simulink model "SOCPIControlBenchmarkRealVarL"  (R2019b)
settings: Solver=FixedStepAuto  StartTime=0.0  StopTime=50000  FixedStep=0.01  RelTol=1e-3
values from neighbouring files (symbols this model uses):
  kio = 0.6    [benchmarkPIDStartRealVarL.m]
  kpo = 1    [benchmarkPIDStartRealVarL.m]
  maxKi = 1    [benchmarkPIDStartRealVarL.m]
  maxKp = 1    [benchmarkPIDStartRealVarL.m]
  minKi = 0.01    [benchmarkPIDStartRealVarL.m]
  minKp = 0.01    [benchmarkPIDStartRealVarL.m]
  N = 100    [benchmarkPIDStartRealVarL.m]
  optimPeriod = 300    [benchmarkPIDStartRealVarL.m]
  OVLim = 2    [benchmarkPIDStartRealVarL.m]
  refAmplitude = 50    [benchmarkPIDStartRealVarL.m]
  refSignalPeriod = optimPeriod    (= 300)    [benchmarkPIDStartRealVarL.m]
  resetThreshold = 0.1    [benchmarkPIDStartRealVarL.m]
undefined symbols (not defined in the file or in its folder): FORandGCNM, sigbuilder_block
libraries: dspmathops x3, simulink x1
(part 1 of 4)
settings Model: Creator=jairo  LastModifiedBy=jairo
settings DataIOCC: ReturnWorkspaceOutputs=off

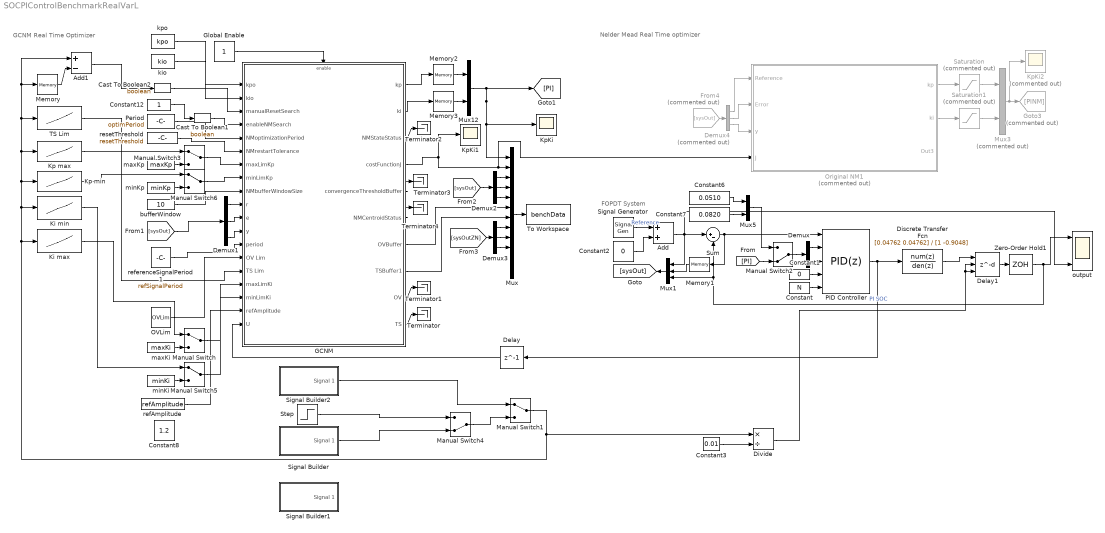
== system SOCPIControlBenchmarkRealVarL ==
  note: FOPDT System
  note: GCNM Real Time Optimizer
  note: Nelder Mead Real Time optimizer
  Add : Sum
  Add1 : Sum  Inputs=+-
  Cast To Boolean1 : DataTypeConversion  OutDataTypeStr=boolean
  Cast To Boolean2 : DataTypeConversion  OutDataTypeStr=boolean
  Constant : Constant  Value=N
  Constant1 : Constant  Value=0
  Constant12 : Constant  OutDataTypeStr=boolean
  Constant2 : Constant  Value=0
  Constant3 : Constant  Value=0.01
  Constant6 : Constant  Value=0.0510
  Constant7 : Constant  Value=0.0820
  Constant8 : Constant  Value=1.2
  Delay : Delay  DelayLength=1
  Delay1 : Delay  DelayLengthSource=Input port  DelayLengthUpperLimit=1000  InitialConditionSource=Input port
      settings: InputPortMap=u0,p1,p4
  Demux : Demux  Outputs=2
  Demux1 : Demux  Outputs=3
  Demux2 : Demux  Outputs=3
  Demux3 : Demux  Outputs=3
  Demux4 : Demux  Commented=on  Outputs=3
  Discrete Transfer Fcn : DiscreteTransferFcn  Numerator=[0.04762 0.04762]  Denominator=[1 -0.9048]
  Divide : Product  Inputs=*/
  From4 : From  Commented=on  GotoTag=sysOut
  GCNM : Subsystem
  Global Enable : Constant
  Goto3 : Goto  Commented=on  GotoTag=PINM
  Ki max : Lookup_n-D  NumberOfTableDimensions=1  BreakpointsForDimension1=[0.1 0.5 1 2 3 4 5 6 7 8 9 10]  UseOneInputPortForAllInputData=on  Table=|  InternalRulePriority=Speed  RndMeth=Simplest  InputSameDT=on
      | [11
      | 1.61
      | 0.9
      | 0.4
      | 0.4
      | 0.3
      | 0.18
      | 0.15
      | 0.12
      | 0.1
      | 0.09
      | 0.07]
  Ki min : Lookup_n-D  NumberOfTableDimensions=1  BreakpointsForDimension1=[0.1 0.5 1 2 3 4 5 6 7 8 9 10]  UseOneInputPortForAllInputData=on  Table=|  InternalRulePriority=Speed  RndMeth=Simplest  InputSameDT=on
      | [1.1
      | 0.41
      | 0.21
      | 0.21
      | 0.11
      | 0.11
      | 0.061
      | 0.06
      | 0.061
      | 0.061
      | 0.061
      | 0.041]
  Kp max : Lookup_n-D  NumberOfTableDimensions=1  BreakpointsForDimension1=[0.1 0.5 1 2 3 4 5 6 7 8 9 10]  UseOneInputPortForAllInputData=on  Table=|  InternalRulePriority=Speed  RndMeth=Simplest  InputSameDT=on
      | [16
      | 3.21
      | 1.8
      | 1
      | 1
      | 0.9
      | 0.68
      | 0.73
      | 0.69
      | 0.67
      | 0.63
      | 0.54]
  Kp min : Lookup_n-D  NumberOfTableDimensions=1  BreakpointsForDimension1=[0.1 0.5 1 2 3 4 5 6 7 8 9 10]  UseOneInputPortForAllInputData=on  Table=|  InternalRulePriority=Speed  RndMeth=Simplest  InputSameDT=on
      | [0.1
      | 0.01
      | 0.01
      | 0.01
      | 0.01
      | 0.01
      | 0.01
      | 0.01
      | 0.01
      | 0.01
      | 0.01
      | 0.01
      | ]
  KpKi : Scope
  KpKi1 : Scope
  KpKi2 : Scope  Commented=on
  Manual Switch{,1,3,5..6} (5 alike) : ManualSwitch
  Manual Switch2 : ManualSwitch  CurrentSetting=0
  Manual Switch4 : ManualSwitch  CurrentSetting=0
  Memory : Memory
  Memory1 : Memory
  Memory2 : Memory  InitialCondition=kpo
  Memory3 : Memory  InitialCondition=kio
  Mux : Mux  Inputs=12
  Mux1 : Mux  Inputs=3
  Mux12 : Mux  Inputs=2
  Mux3 : Mux  Commented=on  Inputs=2
  Mux5 : Mux  Inputs=2
  OVLim : Constant  Value=OVLim
  Original NM1 : Subsystem  Commented=on
  PID Controller : simulink/Continuous/PID Controller  Controller=PID  Form=Parallel  TimeDomain=Discrete-time  SampleTime=0.1  IntegratorMethod=Forward Euler  FilterMethod=Forward Euler  ControllerParametersSource=external  P=1  I=100  D=0  UseFilter=on  N=100  TunerSelectOption=Transfer Function Based (PID Tuner App)  InitialConditionSource=internal  InitialConditionForIntegrator=0  InitialConditionForFilter=0  DifferentiatorICPrevScaledInput=0  ExternalReset=none  TrackingMode=off  Kt=1  LimitOutput=off  UpperSaturationLimit=inf  LowerSaturationLimit=-inf  LinearizeAsGain=on  AntiWindupMode=none  Kb=1  POutMin=[]  POutMax=[]  IOutMin=[]  IOutMax=[]  DOutMin=[]  DOutMax=[]  NOutMin=[]  NOutMax=[]  SumOutMin=[]  SumOutMax=[]  SaturationOutMin=[]  SaturationOutMax=[]  PParamMin=[]  PParamMax=[]  IParamMin=[]  IParamMax=[]  DParamMin=[]  DParamMax=[]  NParamMin=[]  NParamMax=[]  KbParamMin=[]  KbParamMax=[]  KtParamMin=[]  KtParamMax=[]  KbOutMin=[]  KbOutMax=[]  KtOutMin=[]  KtOutMax=[]  IntegratorOutMin=[]  IntegratorOutMax=[]  FilterOutMin=[]  FilterOutMax=[]  SumI1OutMin=[]  SumI1OutMax=[]  SumI2OutMin=[]  SumI2OutMax=[]  SumI3OutMin=[]  SumI3OutMax=[]  SumI4OutMin=[]  SumI4OutMax=[]  SumDOutMin=[]  SumDOutMax=[]  DifferentiatorOutMin=[]  DifferentiatorOutMax=[]  FilterDiffOutCoefMin=[]  FilterDiffOutCoefMax=[]  ReciprocalOutMin=[]  ReciprocalOutMax=[]  SumDenOutMin=[]  SumDenOutMax=[]  SumNumOutMin=[]  SumNumOutMax=[]  DivideOutMin=[]  DivideOutMax=[]  IntegratorContinuousStateAttributes=''  IntegratorStateMustResolveToSignalObject=off  IntegratorRTWStateStorageClass=Auto  FilterContinuousStateAttributes=''  FilterStateMustResolveToSignalObject=off  FilterRTWStateStorageClass=Auto  ParallelPVariant=ExternalParameters  IdealPVariant=Disabled  IVariant=ExternalParameters  DVariant=ExternalParameters  IntegratorVariant=Discrete  SatVariant=Disabled  AWVariant=Passthrough  PCopyVariant=Disabled  TRVariant=Disabled  FdbkBlocksVariant=Forward  IdealPFdbkVariant=Disabled  SatFdbkVariant=Disabled  DerivativeFilterVariant=ForwardEulerFilter  NVariant=ExternalParameters  NCopyVariant=Disabled  FilterICVariant=InternalICsFilter  IntegratorICVariant=InternalICs  ExternalResetVariant=Disabled  TRSumVariant=Passthrough  SumFdbkVariant=Disabled  SumVariant=Sum_PID
  Period : Constant  Value=optimPeriod  OutDataTypeStr=double
  Saturation : Saturate  Commented=on  UpperLimit=maxKp  LowerLimit=minKp
  Saturation1 : Saturate  Commented=on  UpperLimit=maxKi  LowerLimit=minKi
  Signal Generator : SignalGenerator  WaveForm=square  Frequency=1/refSignalPeriod
  Signal Builder : Subsystem  Tag=STV Subsys  LoadFcn=sigbuilder_block('load');  StartFcn=sigbuilder_block('start');  StopFcn=sigbuilder_block('stop');  ClipboardFcn=sigbuilder_block('clipboard');  mask(Sigbuilder block){tuvar=[0:10]}
      mask help: Simulink:masks:SigbuilderBlock_MD
      mask init:
      | if ~strcmp(get_param(bdroot(gcbh),'SimulationStatus'),'stopped') tuvar = sigbuilder_block('maskInit'); end
      settings: CopyFcn=sigbuilder_block('copy');  DeleteFcn=sigbuilder_block('delete');  ModelCloseFcn=sigbuilder_block('modelClose');  PreSaveFcn=sigbuilder_block('preSave');  PauseFcn=sigbuilder_block('pause');  ContinueFcn=sigbuilder_block('continue');  NameChangeFcn=sigbuilder_block('namechange');  OpenFcn=sigbuilder_block('open',[5.4 30.6 1141.2 522.6 ]);  CloseFcn=sigbuilder_block('close');
      mask Display: plot(0, 0, 100, 100,[2, 2, 32, 32, 2], [68, 8, 8, 68, 68],[32, 2], [38, 38], [32, 19, 2],[53, 60, 44], [32, 17, 17, 2],[16, 16, 31, 31]);txt = getActiveGroup(gcbh);text(2, 100, txt,'verticalAlignment', 'top');
  Signal Builder1 : Subsystem  Tag=STV Subsys  LoadFcn=sigbuilder_block('load');  StartFcn=sigbuilder_block('start');  StopFcn=sigbuilder_block('stop');  ClipboardFcn=sigbuilder_block('clipboard');  mask(Sigbuilder block){tuvar=[0:10]}
      mask help: Simulink:masks:SigbuilderBlock_MD
      mask init:
      | if ~strcmp(get_param(bdroot(gcbh),'SimulationStatus'),'stopped') tuvar = sigbuilder_block('maskInit'); end
      settings: CopyFcn=sigbuilder_block('copy');  DeleteFcn=sigbuilder_block('delete');  ModelCloseFcn=sigbuilder_block('modelClose');  PreSaveFcn=sigbuilder_block('preSave');  PauseFcn=sigbuilder_block('pause');  ContinueFcn=sigbuilder_block('continue');  NameChangeFcn=sigbuilder_block('namechange');  OpenFcn=sigbuilder_block('open',[5.4 30.6 1141.2 522.6 ]);  CloseFcn=sigbuilder_block('close');
      mask Display: plot(0, 0, 100, 100,[2, 2, 32, 32, 2], [68, 8, 8, 68, 68],[32, 2], [38, 38], [32, 19, 2],[53, 60, 44], [32, 17, 17, 2],[16, 16, 31, 31]);txt = getActiveGroup(gcbh);text(2, 100, txt,'verticalAlignment', 'top');
  Signal Builder2 : Subsystem  Tag=STV Subsys  LoadFcn=sigbuilder_block('load');  StartFcn=sigbuilder_block('start');  StopFcn=sigbuilder_block('stop');  ClipboardFcn=sigbuilder_block('clipboard');  mask(Sigbuilder block){tuvar=[0:10]}
      mask help: Simulink:masks:SigbuilderBlock_MD
      mask init:
      | if ~strcmp(get_param(bdroot(gcbh),'SimulationStatus'),'stopped') tuvar = sigbuilder_block('maskInit'); end
      settings: CopyFcn=sigbuilder_block('copy');  DeleteFcn=sigbuilder_block('delete');  ModelCloseFcn=sigbuilder_block('modelClose');  PreSaveFcn=sigbuilder_block('preSave');  PauseFcn=sigbuilder_block('pause');  ContinueFcn=sigbuilder_block('continue');  NameChangeFcn=sigbuilder_block('namechange');  OpenFcn=sigbuilder_block('open',[5.4 30.6 1141.2 522.6 ]);  CloseFcn=sigbuilder_block('close');
      mask Display: plot(0, 0, 100, 100,[2, 2, 32, 32, 2], [68, 8, 8, 68, 68],[32, 2], [38, 38], [32, 19, 2],[53, 60, 44], [32, 17, 17, 2],[16, 16, 31, 31]);txt = getActiveGroup(gcbh);text(2, 100, txt,'verticalAlignment', 'top');
  Step : Step  Time=21000  Before=0.1  After=5  SampleTime=0
  Sum : Sum  Inputs=|+-
  TS Lim : Lookup_n-D  NumberOfTableDimensions=1  BreakpointsForDimension1=[0.1 0.5 1 2 3 4 5 6 7 8 9 10]  UseOneInputPortForAllInputData=on  Table=|  InternalRulePriority=Speed  RndMeth=Simplest  InputSameDT=on
      | [40
      | 40
      | 100
      | 100
      | 100
      | 100
      | 100
      | 100
      | 100
      | 100
      | 100
      | 100]
  Terminator{,1..4} (5 alike) : Terminator
  To Workspace : ToWorkspace  VariableName=benchData  SaveFormat=Timeseries  SampleTime=-1
  Zero-Order Hold1 : ZeroOrderHold  SampleTime=-1
  bufferWindow : Constant  Value=10  OutDataTypeStr=uint16
  kio : Constant  Value=kio  OutDataTypeStr=double
  kpo : Constant  Value=kpo  OutDataTypeStr=double
  maxKi : Constant  Value=maxKi  VectorParams1D=off  OutDataTypeStr=double
  maxKp : Constant  Value=maxKp  OutDataTypeStr=double
  minKi : Constant  Value=minKi  OutDataTypeStr=double
  minKp : Constant  Value=minKp  OutDataTypeStr=double
  output : Scope  NumInputPorts=3
  refAmplitude : Constant  Value=refAmplitude  OutDataTypeStr=double
  referenceSignalPeriod1 : Constant  Value=refSignalPeriod
  resetThreshold : Constant  Value=resetThreshold
  wires:
  PID Controller/1 -> Discrete Transfer Fcn/1, Delay/1
  Sum/1 -> Memory1/1, PID Controller/1
  resetThreshold/1 -> GCNM/6(NMrestartTolerance)
  bufferWindow/1 -> GCNM/9(NMbufferWindowSize)
  Cast To Boolean1/1 -> GCNM/4(enableNMSearch)
  kio/1 -> GCNM/2(kio)
  Constant12/1 -> Cast To Boolean1/1
  Global Enable/1 -> GCNM/Enable
  kpo/1 -> GCNM/1(kpo)
  Period/1 -> GCNM/5(NMoptimizationPeriod)
  GCNM/4(costFunctionJ) -> Original NM1/4(J), Mux/2, KpKi1/1
  OVLim/1 -> GCNM/14("  OV Lim")
  Zero-Order Hold1/1 -> output/1, Sum/2, Mux1/3  "PI SOC"
  GCNM/1("  kp") -> Memory2/1
  GCNM/2("  ki") -> Memory3/1
  Mux/1 -> To Workspace/1
  Constant/1 -> PID Controller/5
  Constant1/1 -> PID Controller/4
  Demux/1 -> PID Controller/2
  Demux/2 -> PID Controller/3
  Mux1/1 -> [sysOut]
  [sysOut] -> Demux1/1
  Demux1/1 -> GCNM/10(r)
  Demux1/2 -> GCNM/11("  e")
  Demux1/3 -> GCNM/12("  y")
  [sysOut] -> Demux2/1
  Demux2/1 -> Mux/3
  Demux2/2 -> Mux/4
  Demux2/3 -> Mux/5
  [sysOutZN] -> Demux3/1
  Demux3/1 -> Mux/8
  Demux3/2 -> Mux/9
  Demux3/3 -> Mux/10
  Demux4/2 -> Original NM1/2(Error)
  Demux4/3 -> Original NM1/3(y)
  From4/1 -> Demux4/1
  Demux4/1 -> Original NM1/1(Reference)
  GCNM/10(TS) -> Terminator/1
  GCNM/9(OV) -> Terminator1/1
  GCNM/8(TSBuffer1) -> Mux/7
  GCNM/7(OVBuffer) -> Mux/6
  GCNM/3(NMStateStatus) -> Terminator2/1
  GCNM/5(convergenceThresholdBuffer) -> Terminator3/1
  GCNM/6(NMCentroidStatus) -> Terminator4/1
  Signal Generator/1 -> Add/1  "Reference"
  Constant2/1 -> Add/2
  Add/1 -> output/3, Mux1/1, Sum/1
  refAmplitude/1 -> GCNM/18(refAmplitude)
  Manual Switch2/1 -> Demux/1
  [PI] -> Manual Switch2/2
  Original NM1/2(ki) -> Saturation1/1
  Original NM1/1(kp) -> Saturation/1
  Mux3/1 -> KpKi2/1, Goto3/1
  Mux5/1 -> Manual Switch2/1
  Saturation/1 -> Mux3/1
  Saturation1/1 -> Mux3/2
  Delay/1 -> GCNM/19("  U")
  maxKi/1 -> Manual Switch/2
  Manual Switch/1 -> GCNM/16(maxLimKi)
  Manual Switch3/1 -> GCNM/7(maxLimKp)
  maxKp/1 -> Manual Switch3/2
  Step/1 -> Manual Switch4/1
  Signal Builder/1(Signal 1) -> Manual Switch4/2
  Manual Switch4/1 -> Manual Switch1/2
  minKi/1 -> Manual Switch5/2
  minKp/1 -> Manual Switch6/2
  Manual Switch6/1 -> GCNM/8(minLimKp)
  Manual Switch5/1 -> GCNM/17(minLimKi)
  Divide/1 -> Delay1/3, Delay1/2
  Constant3/1 -> Divide/2
  Discrete Transfer Fcn/1 -> Delay1/1
  Delay1/1 -> Zero-Order Hold1/1
  Mux12/1 -> KpKi/1, Mux/1, [PI]
  Memory1/1 -> Mux1/2
  Memory2/1 -> Mux12/1
  Memory3/1 -> Mux12/2
  Constant7/1 -> Mux5/2
  Constant6/1 -> Mux5/1
  Kp max/1 -> Manual Switch3/1
  Kp min/1 -> Manual Switch6/1
  Ki max/1 -> Manual Switch/1
  Ki min/1 -> Manual Switch5/1
  TS Lim/1 -> GCNM/15(TS Lim)
  referenceSignalPeriod1/1 -> GCNM/13("  period")
  Manual Switch1/1 -> Divide/1, Add1/1, Memory/1, TS Lim/1, Kp max/1, Kp min/1, Ki min/1, Ki max/1
  Memory/1 -> Add1/2
  Add1/1 -> Cast To Boolean2/1
  Cast To Boolean2/1 -> GCNM/3(manualResetSearch)
  Signal Builder2/1(Signal 1) -> Manual Switch1/1

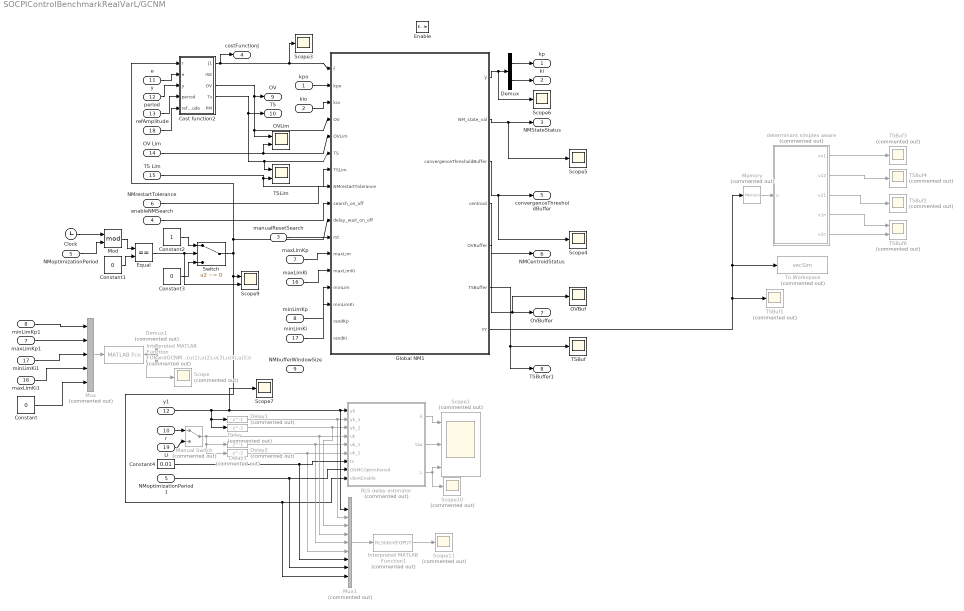
== system SOCPIControlBenchmarkRealVarL/GCNM ==
  kpo : Inport  OutDataTypeStr=double
  kio : Inport  Port=2  OutDataTypeStr=double
  manualResetSearch : Inport  Port=3  OutDataTypeStr=boolean
  enableNMSearch : Inport  Port=4  OutDataTypeStr=boolean
  NMoptimizationPeriod : Inport  Port=5  OutDataTypeStr=double
  NMrestartTolerance : Inport  Port=6
  maxLimKp : Inport  Port=7  OutDataTypeStr=double
  minLimKp : Inport  Port=8  OutDataTypeStr=double
  NMbufferWindowSize : Inport  Port=9  OutDataTypeStr=uint16
  r : Inport  Port=10
  "  e" : Inport  Port=11  OutDataTypeStr=double
  "  y" : Inport  Port=12  OutDataTypeStr=double
  "  period" : Inport  Port=13  OutDataTypeStr=double
  "  OV Lim" : Inport  Port=14  OutDataTypeStr=double
  TS Lim : Inport  Port=15  OutDataTypeStr=double
  maxLimKi : Inport  Port=16  OutDataTypeStr=double
  minLimKi : Inport  Port=17  OutDataTypeStr=double
  refAmplitude : Inport  Port=18  OutDataTypeStr=double
  "  U" : Inport  Port=19  OutDataTypeStr=double
  Enable : EnablePort
  "  y1" : InportShadow  Port=12  OutDataTypeStr=double
  Clock : Clock
  Constant : Constant  Value=0
  Constant1 : Constant  Value=0
  Constant2 : Constant
  Constant3 : Constant  Value=0
  Constant4 : Constant  Value=0.01
  Cost function2 : Subsystem
  Delay : Delay  Commented=on
  Delay1 : Delay  Commented=on  DelayLength=1
  Delay2 : Delay  Commented=on
  Delay3 : Delay  Commented=on  DelayLength=1
  Demux : Demux  Outputs=2
  Demux1 : Demux  Commented=on  Outputs=2
  Equal : RelationalOperator  Operator===  RndMeth=Simplest
  Global NM1 : MATLAB Function  TreatAsAtomicUnit=on
  Interpreted MATLAB Function : MATLABFcn  Commented=on  MATLABFcn=FORandGCNM(u(1),u(2),u(3),u(4),u(5))  OutputDimensions=2
  Interpreted MATLAB Function1 : MATLABFcn  Commented=on  MATLABFcn=RLSIdentFOPDT  OutputDimensions=3
  Manual Switch : ManualSwitch  Commented=on
  Memory : Memory  Commented=on
  Mod : Math  Operator=mod  SignedPower=off  SaturateOnIntegerOverflow=on
  Mux : Mux  Commented=on  Inputs=5
  Mux1 : Mux  Commented=on  Inputs=9
  NMoptimizationPeriod1 : InportShadow  Port=5  OutDataTypeStr=double
  OVBuf : Scope
  OVLim : Scope  NumInputPorts=2
  RLS delay estimator : MATLAB Function  Commented=on  TreatAsAtomicUnit=on  SystemSampleTime=0.01
  Scope : Scope  Commented=on
  Scope1 : Scope  Commented=on  NumInputPorts=3
  Scope10 : Scope  Commented=on
  Scope11 : Scope  Commented=on
  Scope{3..7} (5 alike) : Scope
  Scope9 : Scope  NumInputPorts=2
  Switch : Switch  Criteria=u2 ~= 0
  TSBuf : Scope
  TSBuf{1..4} (4 alike) : Scope  Commented=on
  TSBuf6 : Scope  Commented=on  NumInputPorts=2
  TSLim : Scope  NumInputPorts=2
  To Workspace : ToWorkspace  Commented=on  VariableName=vecSim  SampleTime=-1
  determinant simplex aware : MATLAB Function  Commented=on  TreatAsAtomicUnit=on
  maxLimKi1 : InportShadow  Port=16  OutDataTypeStr=double
  maxLimKp1 : InportShadow  Port=7  OutDataTypeStr=double
  minLimKi1 : InportShadow  Port=17  OutDataTypeStr=double
  minLimKp1 : InportShadow  Port=8  OutDataTypeStr=double
  "  kp" : Outport  OutDataTypeStr=double
  "  ki" : Outport  Port=2  OutDataTypeStr=double
  NMStateStatus : Outport  Port=3  OutDataTypeStr=double
  costFunctionJ : Outport  Port=4  OutDataTypeStr=double
  convergenceThresholdBuffer : Outport  Port=5  OutDataTypeStr=double
  NMCentroidStatus : Outport  Port=6  OutDataTypeStr=double
  OVBuffer : Outport  Port=7  OutDataTypeStr=double
  TSBuffer1 : Outport  Port=8  OutDataTypeStr=double
  OV : Outport  Port=9  OutDataTypeStr=double
  TS : Outport  Port=10  OutDataTypeStr=double
  wires:
  Demux/2 -> "  ki"/1
  Demux/1 -> "  kp"/1
  NMrestartTolerance/1 -> Global NM1/8(NMrestartTolerance)
  manualResetSearch/1 -> Global NM1/11(rst)
  enableNMSearch/1 -> Global NM1/9(search_on_off)
  minLimKp/1 -> Global NM1/14(minLim)
  maxLimKp/1 -> Global NM1/12(maxLim)
  Global NM1/2(NM_state_val) -> Scope5/1, NMStateStatus/1
  Global NM1/3(convergenceThresholdBuffer) -> convergenceThresholdBuffer/1, Scope4/1
  Global NM1/4(centroid) -> NMCentroidStatus/1
  Global NM1/1(y) -> Scope6/1, Demux/1
  kpo/1 -> Global NM1/2(kpo)
  kio/1 -> Global NM1/3(kio)
  Cost function2/3(OV) -> OV/1, Global NM1/4(OV), OVLim/1
  "  y"/1 -> Cost function2/3(y)
  "  e"/1 -> Cost function2/2(e)
  Global NM1/5(OVBuffer) -> OVBuf/1, OVBuffer/1
  "  period"/1 -> Cost function2/4(period)
  "  OV Lim"/1 -> OVLim/2, Global NM1/5(OVLim)
  Cost function2/4(Ts) -> TS/1, Global NM1/6(TS), TSLim/1
  TS Lim/1 -> Global NM1/7(TSLim), TSLim/2
  Global NM1/6(TSBuffer) -> TSBuffer1/1, TSBuf/1
  Cost function2/1(J1) -> Scope3/1, Global NM1/1(f), costFunctionJ/1
  Clock/1 -> Mod/1
  NMoptimizationPeriod/1 -> Mod/2
  Constant1/1 -> Equal/2
  Mod/1 -> Equal/1
  Constant2/1 -> Switch/1
  Constant3/1 -> Switch/3
  Switch/1 -> Mux1/9, RLS delay estimator/9(identEnable), Scope9/1, Cost function2/1(r), Global NM1/10(delay_wait_on_off)
  Equal/1 -> Scope9/2, Switch/2
  maxLimKi/1 -> Global NM1/13(maxLimKi)
  minLimKi/1 -> Global NM1/15(minLimKi)
  refAmplitude/1 -> Cost function2/5(refAmplitude)
  minLimKi1/1 -> Mux/3
  maxLimKi1/1 -> Mux/4
  Mux/1 -> Interpreted MATLAB Function/1
  Interpreted MATLAB Function/1 -> Scope/1, Demux1/1
  maxLimKp1/1 -> Mux/2
  minLimKp1/1 -> Mux/1
  Constant/1 -> Mux/5
  determinant simplex aware/2(v12) -> TSBuf4/1
  Memory/1 -> determinant simplex aware/1(u)
  Global NM1/7(YY) -> TSBuf1/1, To Workspace/1, Memory/1
  determinant simplex aware/5(v2n) -> TSBuf6/2
  determinant simplex aware/3(v21) -> TSBuf2/1
  determinant simplex aware/4(v1n) -> TSBuf6/1
  determinant simplex aware/1(vv1) -> TSBuf3/1
  Delay1/1 -> Mux1/2, RLS delay estimator/2(yk_1)
  Delay/1 -> Mux1/3, RLS delay estimator/3(yk_2)
  "  y1"/1 -> Delay1/1, Delay/1, Scope7/1, Mux1/1, RLS delay estimator/1(yk)
  Delay3/1 -> Mux1/5, RLS delay estimator/5(uk_1)
  Delay2/1 -> RLS delay estimator/6(uk_2), Mux1/6
  NMoptimizationPeriod1/1 -> Mux1/8, RLS delay estimator/8(GNMCOptimPeriod)
  RLS delay estimator/1(k) -> Scope1/1
  RLS delay estimator/2(tau) -> Scope1/2
  RLS delay estimator/3(L) -> Scope1/3, Scope10/1
  Constant4/1 -> Mux1/7, RLS delay estimator/7(ts)
  r/1 -> Manual Switch/1
  "  U"/1 -> Manual Switch/2
  Manual Switch/1 -> Mux1/4, RLS delay estimator/4(uk), Delay2/1, Delay3/1
  Mux1/1 -> Interpreted MATLAB Function1/1
  Interpreted MATLAB Function1/1 -> Scope11/1

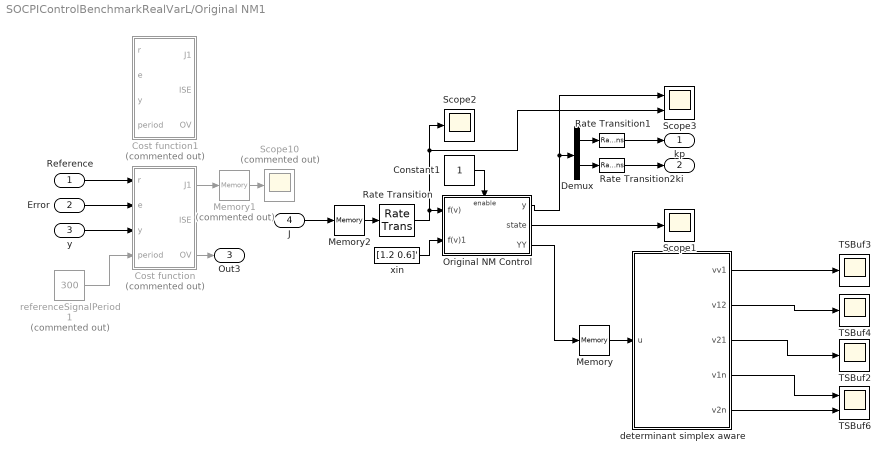
== system SOCPIControlBenchmarkRealVarL/Original NM1 ==
  Reference : Inport
  Error : Inport  Port=2
  y : Inport  Port=3
  J : Inport  Port=4
  Constant1 : Constant
  Cost function : Subsystem  Commented=on
  Cost function1 : Subsystem  Commented=on
  Demux : Demux  Outputs=2
  Memory : Memory
  Memory1 : Memory  Commented=on
  Memory2 : Memory
  Original NM Control : Subsystem
  Rate Transition : RateTransition
  Rate Transition1 : RateTransition  InitialCondition=1
  Rate Transition2 : RateTransition  InitialCondition=100
  Scope1 : Scope
  Scope10 : Scope  Commented=on
  Scope2 : Scope
  Scope3 : Scope  NumInputPorts=2
  TSBuf2 : Scope
  TSBuf3 : Scope
  TSBuf4 : Scope
  TSBuf6 : Scope  NumInputPorts=2
  determinant simplex aware : MATLAB Function  TreatAsAtomicUnit=on
  referenceSignalPeriod1 : Constant  Commented=on  Value=300
  xin : Constant  Value=[1.2 0.6]'
  kp : Outport
  ki : Outport  Port=2
  Out3 : Outport  Port=3
  wires:
  Constant1/1 -> Original NM Control/Enable
  Original NM Control/1(y) -> Scope3/1, Demux/1
  Rate Transition/1 -> Scope2/1, Scope3/2, Original NM Control/1(f(v))
  Demux/2 -> Rate Transition2/1
  xin/1 -> Original NM Control/2(f(v)1)
  y/1 -> Cost function/3(y)
  Original NM Control/2(state) -> Scope1/1
  Demux/1 -> Rate Transition1/1
  Memory2/1 -> Rate Transition/1
  Cost function/3(OV) -> Out3/1
  Memory1/1 -> Scope10/1
  referenceSignalPeriod1/1 -> Cost function/4(period)
  Cost function/1(J1) -> Memory1/1
  Rate Transition1/1 -> kp/1
  Rate Transition2/1 -> ki/1
  Reference/1 -> Cost function/1(r)
  Error/1 -> Cost function/2(e)
  J/1 -> Memory2/1
  determinant simplex aware/2(v12) -> TSBuf4/1
  determinant simplex aware/5(v2n) -> TSBuf6/2
  determinant simplex aware/4(v1n) -> TSBuf6/1
  determinant simplex aware/1(vv1) -> TSBuf3/1
  determinant simplex aware/3(v21) -> TSBuf2/1
  Memory/1 -> determinant simplex aware/1(u)
  Original NM Control/3(YY) -> Memory/1

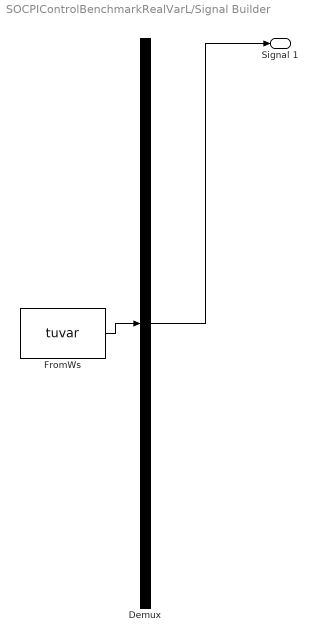
== system SOCPIControlBenchmarkRealVarL/Signal Builder ==
  Demux : Demux  Tag=STV Demux  Outputs=1
  FromWs : FromWorkspace  Tag=STV FromWs  VariableName=tuvar  SampleTime=0
      SigBuilderData=|
      | common.afterFinalStr = 'Extrapolate'
      | common.sampleTime = 0
      | dataSet.timeRange = [0 50000]
      | dataSet.name = 'Group 1'
      | sbobj.Groups.Name = 'Group 1'
      | sbobj.Groups.Signals.Name = 'Signal 1'
      | sbobj.Groups.Signals.XData = [0 12000 12000 21000 21000 36000 36000 50000]
      | sbobj.Groups.Signals.YData = [0.1 0.1 5 5 8 8 3 3]
      | sbobj.Groups.TimeRange = [0 50000]
  Signal 1 : Outport  Tag=STV Outport
  wires:
  Demux/1 -> Signal 1/1
  FromWs/1 -> Demux/1

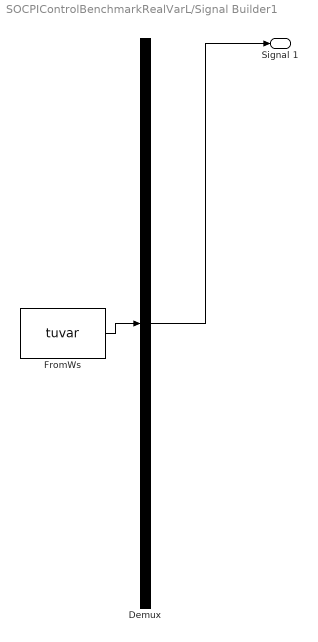
== system SOCPIControlBenchmarkRealVarL/Signal Builder1 ==
  Demux : Demux  Tag=STV Demux  Outputs=1
  FromWs : FromWorkspace  Tag=STV FromWs  VariableName=tuvar  SampleTime=0
      SigBuilderData=|
      | common.afterFinalStr = 'Extrapolate'
      | common.sampleTime = 0
      | dataSet.timeRange = [0 50000]
      | dataSet.name = 'Group 1'
      | sbobj.Groups.Name = 'Group 1'
      | sbobj.Groups.Signals.Name = 'Signal 1'
      | sbobj.Groups.Signals.XData = [0 12000 12000 21000 21000 36000 36000 50000]
      | sbobj.Groups.Signals.YData = [7.98 7.98 5.86 5.86 0.64 0.64 4.2 4.2]
      | sbobj.Groups.TimeRange = [0 50000]
  Signal 1 : Outport  Tag=STV Outport
  wires:
  FromWs/1 -> Demux/1
  Demux/1 -> Signal 1/1

== system SOCPIControlBenchmarkRealVarL/Signal Builder2 ==
  Demux : Demux  Tag=STV Demux  Outputs=1
  FromWs : FromWorkspace  Tag=STV FromWs  VariableName=tuvar  SampleTime=0
      SigBuilderData=|
      | common.afterFinalStr = 'Extrapolate'
      | common.sampleTime = 0
      | dataSet.timeRange = [0 50000]
      | dataSet.name = 'Group 1'
      | sbobj.Groups.Name = 'Group 1'
      | sbobj.Groups.Signals.Name = 'Signal 1'
      | sbobj.Groups.Signals.XData = [0 10050 10050 21000 21000 36000 36000 50000]
      | sbobj.Groups.Signals.YData = [0.1 0.1 9 9 5 5 1 1]
      | sbobj.Groups.TimeRange = [0 50000]
  Signal 1 : Outport  Tag=STV Outport
  wires:
  Demux/1 -> Signal 1/1
  FromWs/1 -> Demux/1

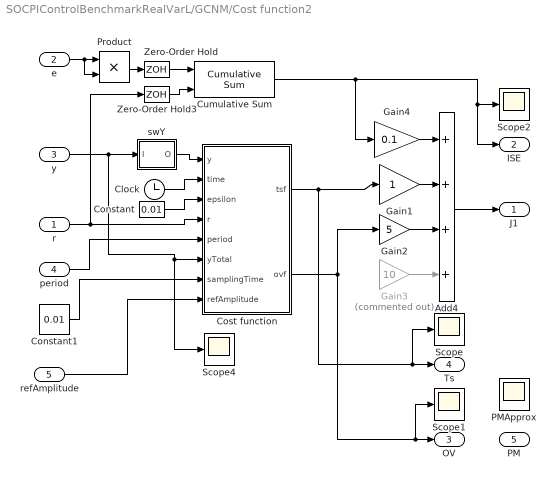
== system SOCPIControlBenchmarkRealVarL/GCNM/Cost function2 ==
  r : Inport
  e : Inport  Port=2
  y : Inport  Port=3
  period : Inport  Port=4
  refAmplitude : Inport  Port=5
  Add4 : Sum  Inputs=++++
  Clock : Clock
  Constant : Constant  Value=0.01
  Constant1 : Constant  Value=0.01
  Cost function : MATLAB Function  TreatAsAtomicUnit=on
  Cumulative Sum : dspmathops/Cumulative Sum  dim=Channels (running sum)  InputProcessing=Columns as channels (frame based)  reset_popup=Falling edge  roundingMode=Floor  overflowMode=off  outputDataTypeStr=Inherit: Same as accumulator  outputMin=[]  outputMax=[]  outputLastDataTypeStr=Inherit: Same as accumulator
      settings: SourceProductName=DSP System Toolbox
  Gain1 : Gain
  Gain2 : Gain  Gain=5
  Gain3 : Gain  Commented=on  Gain=10
  Gain4 : Gain  Gain=0.1
  PMApprox : Scope
  Product : Product
  Scope{,1..2,4} (4 alike) : Scope
  Zero-Order Hold : ZeroOrderHold  SampleTime=-1
  Zero-Order Hold3 : ZeroOrderHold  SampleTime=-1
  swY : Subsystem
  J1 : Outport
  ISE : Outport  Port=2
  OV : Outport  Port=3
  Ts : Outport  Port=4
  PM : Outport  Port=5
  wires:
  Cumulative Sum/1 -> Gain4/1, ISE/1, Scope2/1
  Zero-Order Hold3/1 -> Cumulative Sum/2
  e/1 -> Product/2, Product/1
  Zero-Order Hold/1 -> Cumulative Sum/1
  r/1 -> Zero-Order Hold3/1, Cost function/4(r)
  swY/1(O) -> Cost function/1(y)
  Clock/1 -> Cost function/2(time)
  Product/1 -> Zero-Order Hold/1
  Constant/1 -> Cost function/3(epsilon)
  y/1 -> Scope4/1, Cost function/6(yTotal), swY/1(I)
  Add4/1 -> J1/1
  Gain2/1 -> Add4/3
  period/1 -> Cost function/5(period)
  Constant1/1 -> Cost function/7(samplingTime)
  Gain1/1 -> Add4/2
  refAmplitude/1 -> Cost function/8(refAmplitude)
  Gain3/1 -> Add4/4
  Cost function/1(tsf) -> Gain1/1, Scope/1, Ts/1
  Cost function/2(ovf) -> Gain2/1, Scope1/1, OV/1
  Gain4/1 -> Add4/1

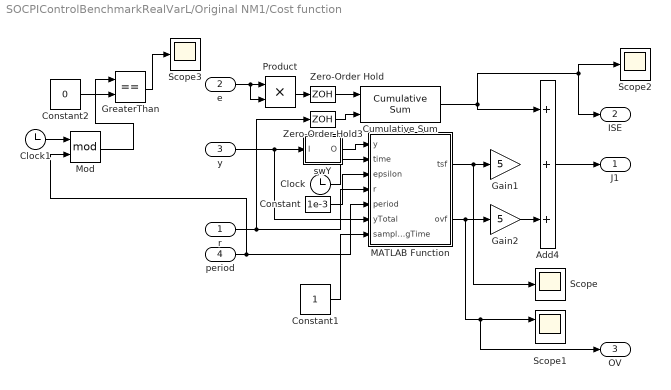
== system SOCPIControlBenchmarkRealVarL/Original NM1/Cost function ==
  r : Inport
  e : Inport  Port=2
  y : Inport  Port=3
  period : Inport  Port=4
  Add4 : Sum  Inputs=+++
  Clock : Clock
  Clock1 : Clock
  Constant : Constant  Value=1e-3
  Constant1 : Constant
  Constant2 : Constant  Value=0
  Cumulative Sum : dspmathops/Cumulative Sum  dim=Channels (running sum)  InputProcessing=Columns as channels (frame based)  reset_popup=Falling edge  roundingMode=Floor  overflowMode=off  outputDataTypeStr=Inherit: Same as accumulator  outputMin=[]  outputMax=[]  outputLastDataTypeStr=Inherit: Same as accumulator
      settings: SourceProductName=DSP System Toolbox
  Gain1 : Gain  Gain=5
  Gain2 : Gain  Gain=5
  GreaterThan : RelationalOperator  Operator===  OutDataTypeStr=boolean  RndMeth=Simplest
  MATLAB Function : MATLAB Function  TreatAsAtomicUnit=on
  Mod : Math  Operator=mod  SignedPower=off  SaturateOnIntegerOverflow=on
  Product : Product
  Scope : Scope
  Scope1 : Scope  NumInputPorts=2
  Scope2 : Scope
  Scope3 : Scope
  Zero-Order Hold : ZeroOrderHold  SampleTime=-1
  Zero-Order Hold3 : ZeroOrderHold  SampleTime=-1
  swY : Subsystem
  J1 : Outport
  ISE : Outport  Port=2
  OV : Outport  Port=3
  wires:
  Cumulative Sum/1 -> Add4/1, ISE/1, Scope2/1
  Zero-Order Hold3/1 -> Cumulative Sum/2
  e/1 -> Product/2, Product/1
  MATLAB Function/1(tsf) -> Scope/1, Gain1/1
  Zero-Order Hold/1 -> Cumulative Sum/1
  r/1 -> Zero-Order Hold3/1, MATLAB Function/4(r)
  MATLAB Function/2(ovf) -> OV/1, Scope1/1, Gain2/1
  swY/1(O) -> MATLAB Function/1(y)
  Clock/1 -> MATLAB Function/2(time)
  Product/1 -> Zero-Order Hold/1
  Constant/1 -> MATLAB Function/3(epsilon)
  y/1 -> MATLAB Function/6(yTotal), swY/1(I)
  Add4/1 -> J1/1
  Gain2/1 -> Add4/3
  Constant1/1 -> MATLAB Function/7(samplingTime)
  Clock1/1 -> Mod/1
  Mod/1 -> GreaterThan/1
  period/1 -> MATLAB Function/5(period), Mod/2
  GreaterThan/1 -> Scope3/1
  Constant2/1 -> GreaterThan/2

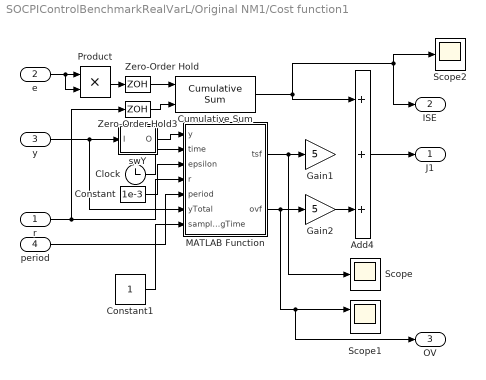
== system SOCPIControlBenchmarkRealVarL/Original NM1/Cost function1 ==
  r : Inport
  e : Inport  Port=2
  y : Inport  Port=3
  period : Inport  Port=4
  Add4 : Sum  Inputs=+++
  Clock : Clock
  Constant : Constant  Value=1e-3
  Constant1 : Constant
  Cumulative Sum : dspmathops/Cumulative Sum  dim=Channels (running sum)  InputProcessing=Columns as channels (frame based)  reset_popup=Falling edge  roundingMode=Floor  overflowMode=off  outputDataTypeStr=Inherit: Same as accumulator  outputMin=[]  outputMax=[]  outputLastDataTypeStr=Inherit: Same as accumulator
      settings: SourceProductName=DSP System Toolbox
  Gain1 : Gain  Gain=5
  Gain2 : Gain  Gain=5
  MATLAB Function : MATLAB Function  TreatAsAtomicUnit=on
  Product : Product
  Scope : Scope
  Scope1 : Scope  NumInputPorts=2
  Scope2 : Scope
  Zero-Order Hold : ZeroOrderHold  SampleTime=-1
  Zero-Order Hold3 : ZeroOrderHold  SampleTime=-1
  swY : Subsystem
  J1 : Outport
  ISE : Outport  Port=2
  OV : Outport  Port=3
  wires:
  Constant1/1 -> MATLAB Function/7(samplingTime)
  period/1 -> MATLAB Function/5(period)
  Gain2/1 -> Add4/3
  Add4/1 -> J1/1
  y/1 -> swY/1(I), MATLAB Function/6(yTotal)
  Constant/1 -> MATLAB Function/3(epsilon)
  Product/1 -> Zero-Order Hold/1
  Clock/1 -> MATLAB Function/2(time)
  swY/1(O) -> MATLAB Function/1(y)
  MATLAB Function/2(ovf) -> Gain2/1, Scope1/1, OV/1
  r/1 -> MATLAB Function/4(r), Zero-Order Hold3/1
  Zero-Order Hold/1 -> Cumulative Sum/1
  MATLAB Function/1(tsf) -> Gain1/1, Scope/1
  e/1 -> Product/1, Product/2
  Zero-Order Hold3/1 -> Cumulative Sum/2
  Cumulative Sum/1 -> Scope2/1, ISE/1, Add4/1

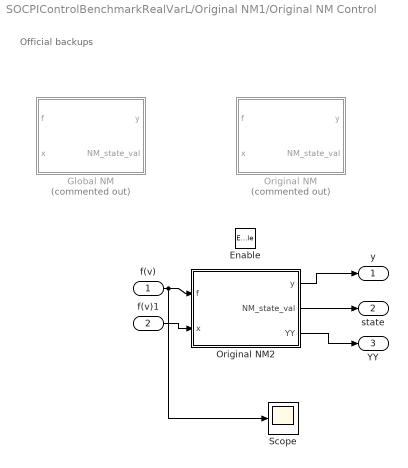
== system SOCPIControlBenchmarkRealVarL/Original NM1/Original NM Control ==
  note: Official backups
  f(v) : Inport
  f(v)1 : Inport  Port=2
  Enable : EnablePort
  Global NM : MATLAB Function  Commented=on  TreatAsAtomicUnit=on
  Original NM : MATLAB Function  Commented=on  TreatAsAtomicUnit=on
  Original NM2 : MATLAB Function  TreatAsAtomicUnit=on  SystemSampleTime=300
  Scope : Scope
  y : Outport
  state : Outport  Port=2
  YY : Outport  Port=3
  wires:
  f(v)/1 -> Scope/1, Original NM2/1(f)
  Original NM2/1(y) -> y/1
  Original NM2/2(NM_state_val) -> state/1
  f(v)1/1 -> Original NM2/2(x)
  Original NM2/3(YY) -> YY/1

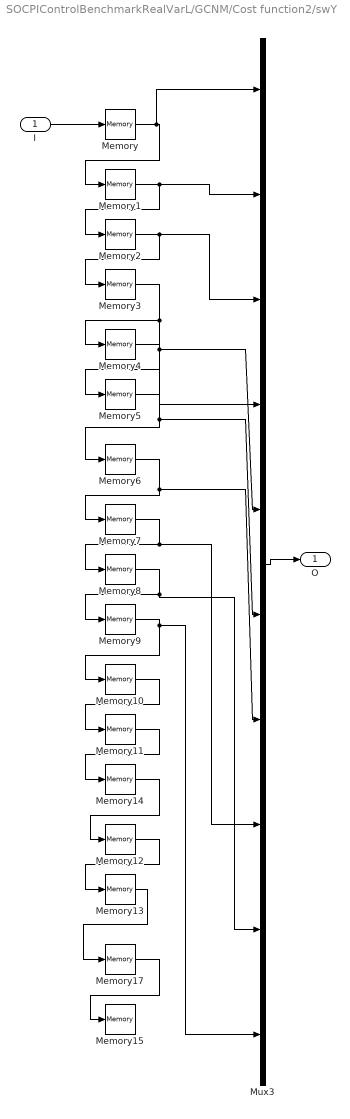
== system SOCPIControlBenchmarkRealVarL/GCNM/Cost function2/swY ==
  I : Inport
  Memory{,1..15,17} (17 alike) : Memory
  Mux3 : Mux  Inputs=10
  O : Outport
  wires:
  Memory11/1 -> Memory14/1
  Memory14/1 -> Memory12/1
  Memory12/1 -> Memory13/1
  Memory13/1 -> Memory17/1
  Memory5/1 -> Memory6/1, Mux3/6
  Memory4/1 -> Memory5/1, Mux3/5
  Mux3/1 -> O/1
  Memory9/1 -> Memory10/1, Mux3/10
  Memory3/1 -> Memory4/1, Mux3/4
  Memory6/1 -> Memory7/1, Mux3/7
  Memory1/1 -> Memory2/1, Mux3/2
  Memory10/1 -> Memory11/1
  Memory2/1 -> Memory3/1, Mux3/3
  I/1 -> Memory/1
  Memory8/1 -> Memory9/1, Mux3/9
  Memory/1 -> Memory1/1, Mux3/1
  Memory7/1 -> Memory8/1, Mux3/8
  Memory17/1 -> Memory15/1

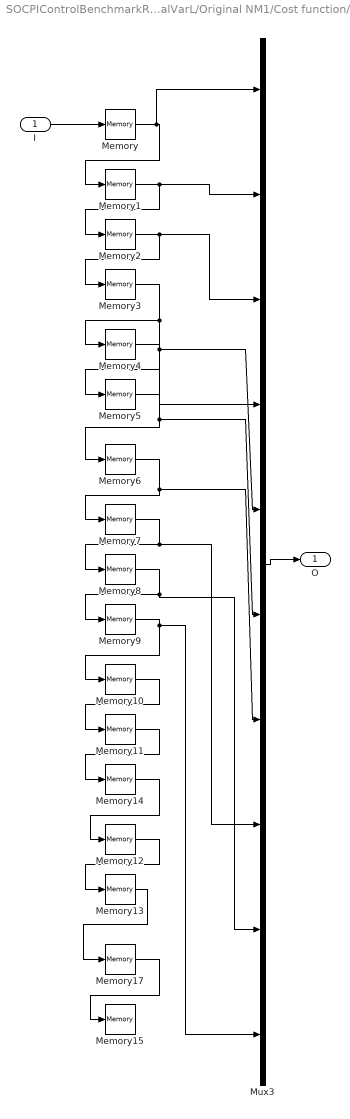
== system SOCPIControlBenchmarkRealVarL/Original NM1/Cost function/swY ==
  I : Inport
  Memory{,1..15,17} (17 alike) : Memory
  Mux3 : Mux  Inputs=10
  O : Outport
  wires:
  Memory11/1 -> Memory14/1
  Memory14/1 -> Memory12/1
  Memory12/1 -> Memory13/1
  Memory13/1 -> Memory17/1
  Memory5/1 -> Memory6/1, Mux3/6
  Memory4/1 -> Memory5/1, Mux3/5
  Mux3/1 -> O/1
  Memory9/1 -> Memory10/1, Mux3/10
  Memory3/1 -> Memory4/1, Mux3/4
  Memory6/1 -> Memory7/1, Mux3/7
  Memory1/1 -> Memory2/1, Mux3/2
  Memory10/1 -> Memory11/1
  Memory2/1 -> Memory3/1, Mux3/3
  I/1 -> Memory/1
  Memory8/1 -> Memory9/1, Mux3/9
  Memory/1 -> Memory1/1, Mux3/1
  Memory7/1 -> Memory8/1, Mux3/8
  Memory17/1 -> Memory15/1

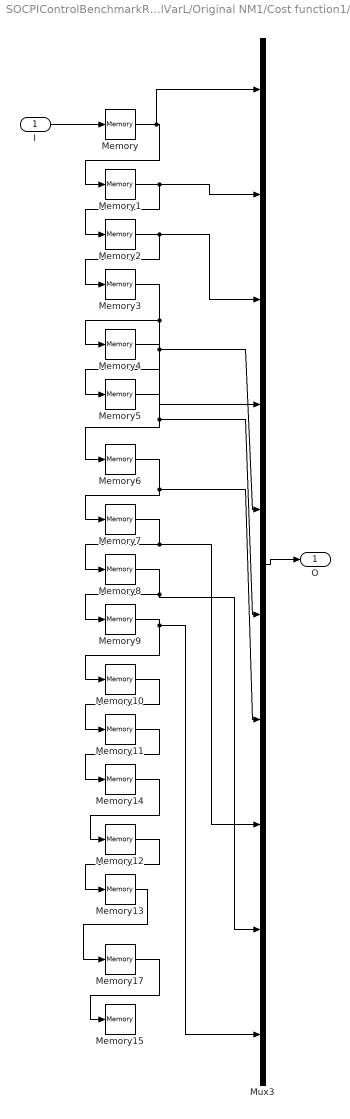
== system SOCPIControlBenchmarkRealVarL/Original NM1/Cost function1/swY ==
  I : Inport
  Memory{,1..15,17} (17 alike) : Memory
  Mux3 : Mux  Inputs=10
  O : Outport
  wires:
  Memory17/1 -> Memory15/1
  Memory7/1 -> Mux3/8, Memory8/1
  Memory/1 -> Mux3/1, Memory1/1
  Memory8/1 -> Mux3/9, Memory9/1
  I/1 -> Memory/1
  Memory2/1 -> Mux3/3, Memory3/1
  Memory10/1 -> Memory11/1
  Memory1/1 -> Mux3/2, Memory2/1
  Memory6/1 -> Mux3/7, Memory7/1
  Memory3/1 -> Mux3/4, Memory4/1
  Memory9/1 -> Mux3/10, Memory10/1
  Mux3/1 -> O/1
  Memory4/1 -> Mux3/5, Memory5/1
  Memory5/1 -> Mux3/6, Memory6/1
  Memory13/1 -> Memory17/1
  Memory12/1 -> Memory13/1
  Memory14/1 -> Memory12/1
  Memory11/1 -> Memory14/1

== matlab function SOCPIControlBenchmarkRealVarL/GCNM/RLS delay estimator ==
  data: yk input; k output; yk_1 input; yk_2 input; uk input; uk_1 input; uk_2 input; tau output; L output; ts input; GNMCOptimPeriod input; identEnable input
function [k,tau,L] = RLSIdentFOPDT(yk,yk_1,yk_2,uk,uk_1,uk_2,ts,GNMCOptimPeriod,identEnable)
persistent y y_1 y_2 u u_1 u_2 counter
persistent k_RLS tau_RLS L_RLS

%RT identification arrays initialization
if isempty(y)
    y=zeros(1,GNMCOptimPeriod/ts);
    y_1=zeros(1,GNMCOptimPeriod/ts);
    y_2=zeros(1,GNMCOptimPeriod/ts);
    u=zeros(1,GNMCOptimPeriod/ts);
    u_1=zeros(1,GNMCOptimPeriod/ts);
    u_2=zeros(1,GNMCOptimPeriod/ts);
    counter=1;      
    k_RLS=0; tau_RLS=0; L_RLS=0;
end

if identEnable>0.5
%     tau1=y;
    tau1=y(round(length(y))/2:end-1000);
    tau1(tau1<0)=0;
%     tau1(1)=0;
    y_11 = circshift(tau1,[1,1]); y_11(1)=0;
    y_22 = circshift(tau1,[1,2]); y_22(1:2)=0;
%     u_k=u;
    u_k  = u(round(length(u))/2:end-1000);
    u_11 = circshift(u_k,[1,1]); u_11(1)=0;
    u_22 = circshift(u_k,[1,2]); u_22(1:2)=0;
    
%     tau1=y(round(length(y)/2):end-1000);
    m=length(tau1); 
    %phi matrix
    fi11=u_k; fi12=u_11; fi13=u_22;  fi14=y_11; fi15=y_22; 
    fi=[fi11', fi12', fi13', fi14', fi15'];
    %MIMO RLS algorithm
    theta=mincuadm(tau1,fi,m,5,1);
    T=ts;
    ABC_RLS=2/(theta(2));
    A_RLS=-(theta(4)*ABC_RLS+2)/2;
%     B_RLS=ABC_RLS-A_RLS-1;
    L_RLS=T*(theta(3)-theta(1))/(theta(3)+theta(1));
    tau_RLS= A_RLS/(L_RLS*0.5*(2/T)^2);
    k_RLS= (theta(3)*ABC_RLS) /((T+L_RLS)/T);
    k=k_RLS; tau=tau_RLS; L=L_RLS;
    
%     data=iddata(tau1,u,ts);
%     m = procest(data,'P1D')
    
    %arrays cleaning
    y=zeros(1,GNMCOptimPeriod/ts);
    y_1=zeros(1,GNMCOptimPeriod/ts);
    y_2=zeros(1,GNMCOptimPeriod/ts);
    u=zeros(1,GNMCOptimPeriod/ts);
    u_1=zeros(1,GNMCOptimPeriod/ts);
    u_2=zeros(1,GNMCOptimPeriod/ts);
    
    
    counter=1;
else
    y(counter)=yk;
    y_1(counter)=yk_1;
    y_2(counter)=yk_2;
    u(counter)=uk;
    u_1(counter)=uk_1;
    u_2(counter)=uk_2;
    
    counter=counter+1;
    k=k_RLS; tau=tau_RLS; L=L_RLS;
end
